simulink model "joystick"  (R2014b)
settings: Solver=ode45  StartTime=0.0  StopTime=inf  RelTol=1e-3
libraries: vrlib x1, slrtlib x1
settings Model: Creator=wmartin  LastModifiedBy=wmartin

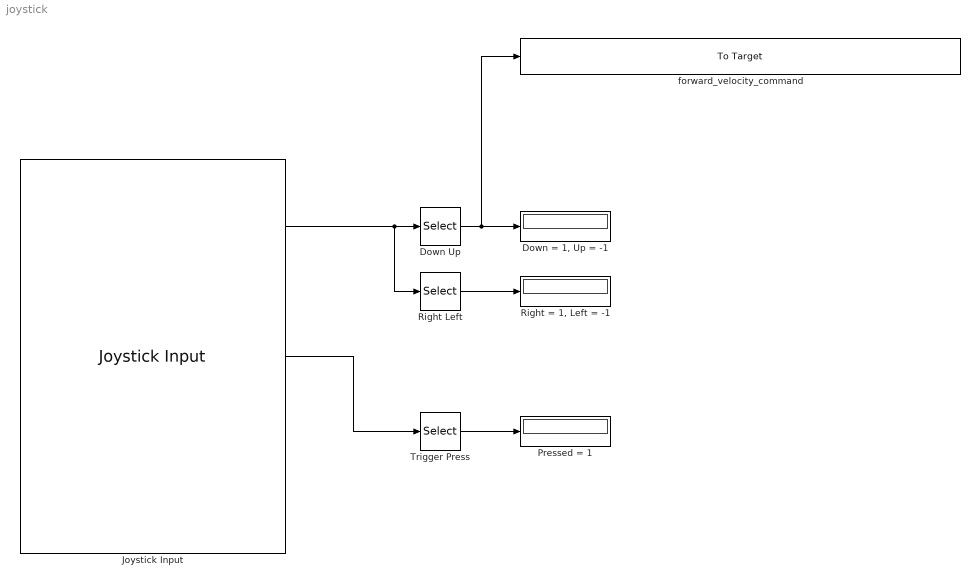
== system joystick ==
  "Down = 1, Up = -1" : Display
  Down Up : Selector  InputPortWidth=4  Indices=[2]
  Joystick Input : vrlib/Joystick Input  joyid=1  adjustports=on  forcefeed=off
  Pressed = 1 : Display
  "Right = 1, Left = -1" : Display
  Right Left : Selector  InputPortWidth=4  Indices=[1]
  Trigger Press : Selector  InputPortWidth=12  Indices=[1]
  forward_velocity_command : slrtlib/Displays and Logging/To Target   appname=linearized_smm_with_lqr_2d  blockpath=Control/Behavior Control/Primary Leg Behavior/Running/forward_velocity_command  paramname=Value  isdefault=on
  wires:
  Joystick Input/1 -> Right Left/1, Down Up/1
  Right Left/1 -> "Right = 1, Left = -1"/1
  Joystick Input/2 -> Trigger Press/1
  Trigger Press/1 -> Pressed = 1/1
  Down Up/1 -> forward_velocity_command/1, "Down = 1, Up = -1"/1
